simulink model "rising_hil"  (R2019b)
settings: Solver=FixedStepAuto  StartTime=0.0  StopTime=30  FixedStep=1  RelTol=1e-3
model workspace (MAT data in the model file):
  ALS_mode = Simulink.Signal
  ALS_mode.DataType = 'Enum: angle'
  ALS_mode.Dimensions = -1
  ALS_mode.DimensionsMode = 'auto'
  ALS_mode.Complexity = 'auto'
  ALS_mode.SampleTime = -1
  ALS_mode.SamplingMode = 'auto'
  ALS_mode_off = Simulink.Parameter
  ALS_mode_off.DataType = 'Enum: angle'
  ALS_mode_off.Dimensions = [0 0]
  ALS_mode_on = Simulink.Parameter
  ALS_mode_on.DataType = 'Enum: angle'
  ALS_mode_on.Dimensions = [0 0]
  Angle = Simulink.Signal
  Angle.DataType = 'uint8'
  Angle.Dimensions = -1
  Angle.DimensionsMode = 'auto'
  Angle.Complexity = 'auto'
  Angle.SampleTime = -1
  Angle.SamplingMode = 'auto'
  Carangle = Simulink.Parameter
  Carangle.Value = 25
  Carangle.DataType = 'uint8'
  Carangle.Dimensions = [1 1]
  Darkness_mode = Simulink.Signal
  Darkness_mode.DataType = 'Enum: angle'
  Darkness_mode.Dimensions = -1
  Darkness_mode.DimensionsMode = 'auto'
  Darkness_mode.Complexity = 'auto'
  Darkness_mode.SampleTime = -1
  Darkness_mode.SamplingMode = 'auto'
  Darkness_mode_off = Simulink.Parameter
  Darkness_mode_off.DataType = 'Enum: angle'
  Darkness_mode_off.Dimensions = [0 0]
  Darkness_mode_on = Simulink.Parameter
  Darkness_mode_on.DataType = 'Enum: angle'
  Darkness_mode_on.Dimensions = [0 0]
  Headlight_off = Simulink.Parameter
  Headlight_off.DataType = 'Enum: angle'
  Headlight_off.Dimensions = [0 0]
  High_Beam = Simulink.Parameter
  High_Beam.DataType = 'Enum: angle'
  High_Beam.Dimensions = [0 0]
  Ignition_off = Simulink.Parameter
  Ignition_off.DataType = 'angle'
  Ignition_off.Dimensions = [0 0]
  Ignition_on = Simulink.Parameter
  Ignition_on.DataType = 'Enum: angle'
  Ignition_on.Dimensions = [0 0]
  Ignitition = Simulink.Signal
  Ignitition.DataType = 'Enum:angle'
  Ignitition.Dimensions = -1
  Ignitition.DimensionsMode = 'auto'
  Ignitition.Complexity = 'auto'
  Ignitition.SampleTime = -1
  Ignitition.SamplingMode = 'auto'
  Low_Beam = Simulink.Parameter
  Low_Beam.DataType = 'Enum: angle'
  Low_Beam.Dimensions = [0 0]
  Time = Simulink.Parameter
  Time.Value = 2
  Time.DataType = 'uint8'
  Time.Dimensions = [1 1]
values from neighbouring files (symbols this model uses):
  Carangle = 25.0    [ALS_Project_dd.sldd]    (also in Car_Angle.m = Simulink.Parameter)
  Time = 2.0    [ALS_Project_dd.sldd]    (also in Car_Angle.m = Simulink.Parameter)
undefined symbols (not defined in the file or in its folder): angle, sigbuilder_block
libraries: simulink x6
settings Model: DataDictionary=Rising_hill_Data_Dictionary_2.sldd  OrderedModelArguments=off  Creator=Pravin  LastModifiedBy=Pravin
settings OptimizationCC: DefaultParameterBehavior=Inlined  EnhancedBackFolding=on  PassReuseOutputArgsAs=Individual arguments  ZeroExternalMemoryAtStartup=off  ZeroInternalMemoryAtStartup=off  OptimizeBlockOrder=speed  DifferentSizesBufferReuse=on  OptimizationCustomize=off  EfficientTunableParamExpr=on
settings DebuggingCC: ParameterTunabilityLossMsg=error
settings SFSimCC: MATLABDynamicMemAlloc=off
settings RTWCC: SystemTargetFile=ert.tlc  GenCodeOnly=on  TemplateMakefile=ert_default_tmf  GenerateReport=on  IncludeHyperlinkInReport=on  LaunchReport=on  GenerateTraceInfo=on  GenerateTraceReport=on  GenerateTraceReportSl=on  GenerateTraceReportSf=on  GenerateTraceReportEml=on
settings CodeAppCC: ForceParamTrailComments=on  IgnoreCustomStorageClasses=off  OperatorAnnotations=on  SimulinkDataObjDesc=on  SFDataObjDesc=on  InsertBlockDesc=on
settings ERTTargetCC: TargetLangStandard=C99 (ISO)  GenerateSampleERTMain=on  InlinedParameterPlacement=NonHierarchical  ERTCustomFileTemplate=example_file_process.tlc
settings ConfigComp: CovMetricSettings=dcmwe

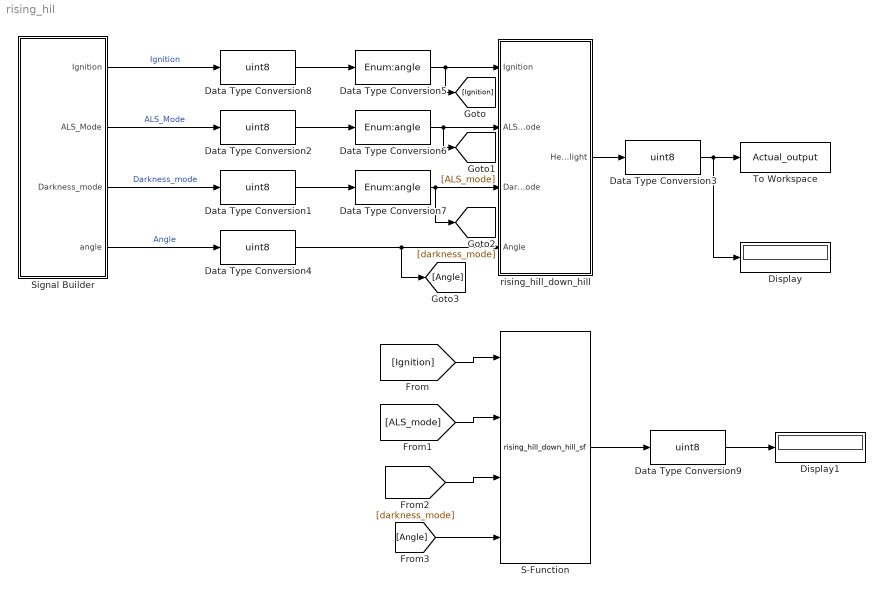
== system rising_hil ==
  Data Type Conversion{1..2,4,8} (4 alike) : DataTypeConversion  OutDataTypeStr=uint8  SaturateOnIntegerOverflow=on
  Data Type Conversion3 : DataTypeConversion  OutDataTypeStr=uint8
  Data Type Conversion5 : DataTypeConversion  OutDataTypeStr=Enum:angle  SaturateOnIntegerOverflow=on
  Data Type Conversion6 : DataTypeConversion  OutDataTypeStr=Enum:angle  SaturateOnIntegerOverflow=on
  Data Type Conversion7 : DataTypeConversion  OutDataTypeStr=Enum:angle  SaturateOnIntegerOverflow=on
  Data Type Conversion9 : DataTypeConversion  OutDataTypeStr=uint8
  Display : Display
  Display1 : Display
  S-Function : S-Function  FunctionName=rising_hill_down_hill_sf  SFunctionDeploymentMode=off  EnableBusSupport=off  SFcnStateName=DWORK0
      settings: SFcnIsStateOwnerBlock=on
  Signal Builder : Subsystem  Tag=STV Subsys  LoadFcn=sigbuilder_block('load',[437.6 153 550.4 359.25 ]);  StartFcn=sigbuilder_block('start');  StopFcn=sigbuilder_block('stop');  ClipboardFcn=sigbuilder_block('clipboard');  mask(Sigbuilder block){tuvar=[0:10]}
      mask help: Simulink:masks:SigbuilderBlock_MD
      mask init:
      | if ~strcmp(get_param(bdroot(gcbh),'SimulationStatus'),'stopped') tuvar = sigbuilder_block('maskInit'); end
      settings: CopyFcn=sigbuilder_block('copy');  DeleteFcn=sigbuilder_block('delete');  ModelCloseFcn=sigbuilder_block('modelClose');  PreSaveFcn=sigbuilder_block('preSave');  PauseFcn=sigbuilder_block('pause');  ContinueFcn=sigbuilder_block('continue');  NameChangeFcn=sigbuilder_block('namechange');  OpenFcn=sigbuilder_block('open',[437.6 153 550.4 359.25 ]);  CloseFcn=sigbuilder_block('close');
      mask Display: plot(0, 0, 100, 100,[2, 2, 32, 32, 2], [68, 8, 8, 68, 68],[32, 2], [38, 38], [32, 19, 2],[53, 60, 44], [32, 17, 17, 2],[16, 16, 31, 31]);txt = getActiveGroup(gcbh);text(2, 100, txt,'verticalAlignment', 'top');
  To Workspace : ToWorkspace  VariableName=Actual_output  SaveFormat=Timeseries  SampleTime=-1
  rising_hill_down_hill : Subsystem  TreatAsAtomicUnit=on
  wires:
  Signal Builder/4(angle) -> Data Type Conversion4/1  "Angle"
  rising_hill_down_hill/1("Headlight ") -> Data Type Conversion3/1
  Signal Builder/3(Darkness_mode) -> Data Type Conversion1/1  "Darkness_mode"
  Signal Builder/1(Ignition) -> Data Type Conversion8/1  "Ignition"
  Data Type Conversion5/1 -> [Ignition], rising_hill_down_hill/1(Ignition)
  Data Type Conversion6/1 -> rising_hill_down_hill/2("ALS_mode "), [ALS_mode]
  Data Type Conversion3/1 -> Display/1, To Workspace/1
  Data Type Conversion4/1 -> rising_hill_down_hill/4("Angle "), [Angle]
  Data Type Conversion7/1 -> rising_hill_down_hill/3("Darkness_mode "), [darkness_mode]
  Signal Builder/2(ALS_Mode) -> Data Type Conversion2/1  "ALS_Mode"
  Data Type Conversion1/1 -> Data Type Conversion7/1
  Data Type Conversion2/1 -> Data Type Conversion6/1
  Data Type Conversion8/1 -> Data Type Conversion5/1
  [Ignition] -> S-Function/1
  [ALS_mode] -> S-Function/2
  [darkness_mode] -> S-Function/3
  [Angle] -> S-Function/4
  S-Function/1 -> Data Type Conversion9/1
  Data Type Conversion9/1 -> Display1/1

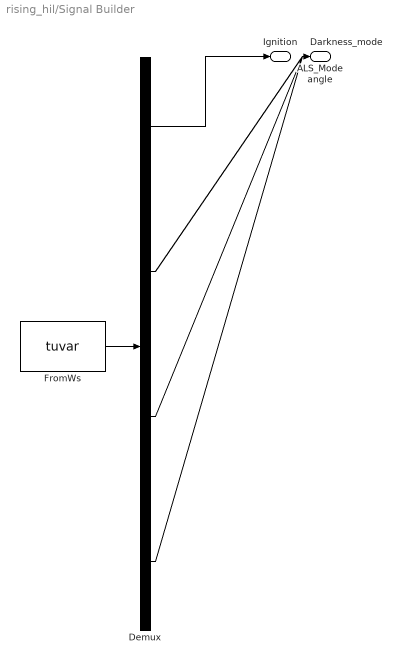
== system rising_hil/Signal Builder ==
  Demux : Demux  Tag=STV Demux
  FromWs : FromWorkspace  Tag=STV FromWs  VariableName=tuvar  SampleTime=0
      SigBuilderData=|
      | common.afterFinalStr = 'Extrapolate'
      | common.sampleTime = 0
      | dataSet.timeRange = [0 10]
      | dataSet.name = 'Sheet1'
      | sbobj.Name = 'Signal Builder'
      | sbobj.Groups.Name = 'Sheet1'
      | sbobj.Groups.Signals(1).Name = 'Ignition'
      | sbobj.Groups.Signals(1).XData = [0 1 2 3 4 5 6 7 8 9 10]
      | sbobj.Groups.Signals(1).YData = [2 3 2 2 2 2 3 3 2 2 2]
      | sbobj.Groups.Signals(2).Name = 'ALS_Mode'
      | sbobj.Groups.Signals(2).XData = [0 1 2 3 4 5 6 7 8 9 10]
      | sbobj.Groups.Signals(2).YData = [4 4 5 4 4 4 5 5 4 4 4]
      | sbobj.Groups.Signals(3).Name = 'Darkness_mode'
      | sbobj.Groups.Signals(3).XData = [0 1 2 3 4 5 6 7 8 9 10]
      | sbobj.Groups.Signals(3).YData = [6 6 6 7 6 6 7 7 6 6 6]
      | sbobj.Groups.Signals(4).Name = 'angle'
      | sbobj.Groups.Signals(4).XData = [0 1 2 3 4 5 6 7 8 9 10]
      | sbobj.Groups.Signals(4).YData = [20 25 26 25 25 25 20 26 26 22 0]
  Ignition : Outport  Tag=STV Outport
  ALS_Mode : Outport  Tag=STV Outport  Port=2
  Darkness_mode : Outport  Tag=STV Outport  Port=3
  angle : Outport  Tag=STV Outport  Port=4
  wires:
  Demux/1 -> Ignition/1
  FromWs/1 -> Demux/1
  Demux/2 -> ALS_Mode/1
  Demux/3 -> Darkness_mode/1
  Demux/4 -> angle/1

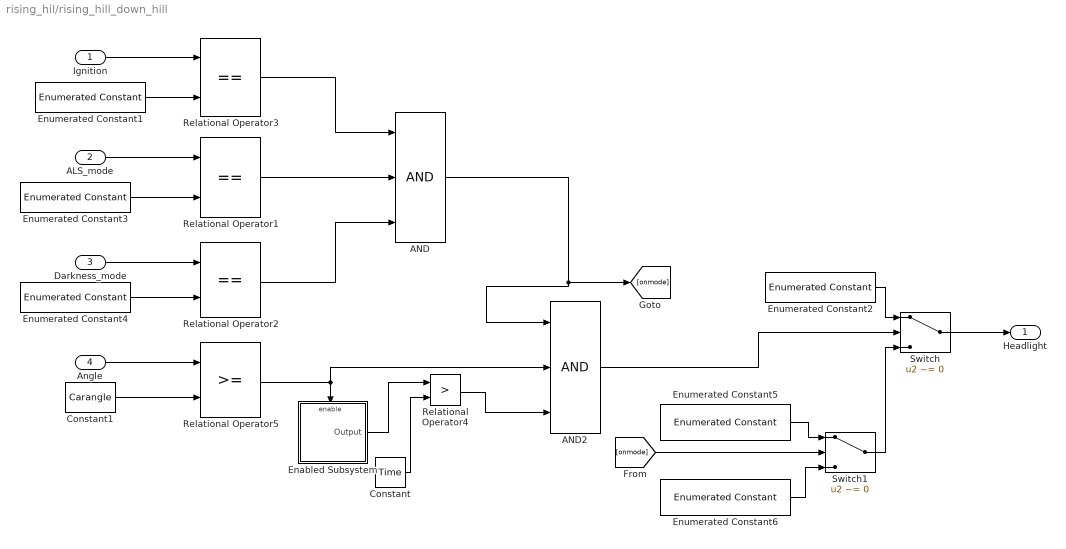
== system rising_hil/rising_hill_down_hill ==
  Ignition : Inport
  "ALS_mode " : Inport  Port=2
  "Darkness_mode " : Inport  Port=3
  "Angle " : Inport  Port=4
  AND : Logic  Inputs=3  AllPortsSameDT=off  OutDataTypeStr=boolean
  AND2 : Logic  Inputs=3  AllPortsSameDT=off  OutDataTypeStr=boolean
  Constant : Constant  Value=Time
  Constant1 : Constant  Value=Carangle
  Enabled Subsystem : Subsystem  TreatAsAtomicUnit=on
  Enumerated Constant1 : simulink/Sources/Enumerated Constant  OutDataTypeStr=Enum:angle  Value=angle.Ignition_on  SampleTime=inf
      settings: SourceProductName=Simulink
  Enumerated Constant2 : simulink/Sources/Enumerated Constant  OutDataTypeStr=Enum:angle  Value=angle.High_Beam  SampleTime=inf
      settings: SourceProductName=Simulink
  Enumerated Constant3 : simulink/Sources/Enumerated Constant  OutDataTypeStr=Enum:angle  Value=angle.ALS_mode_on  SampleTime=inf
      settings: SourceProductName=Simulink
  Enumerated Constant4 : simulink/Sources/Enumerated Constant  OutDataTypeStr=Enum:angle  Value=angle.Darkness_mode_on  SampleTime=inf
      settings: SourceProductName=Simulink
  Enumerated Constant5 : simulink/Sources/Enumerated Constant  OutDataTypeStr=Enum:angle  Value=angle.Low_Beam  SampleTime=inf
      settings: SourceProductName=Simulink
  Enumerated Constant6 : simulink/Sources/Enumerated Constant  OutDataTypeStr=Enum:angle  Value=angle.Headlight_off  SampleTime=inf
      settings: SourceProductName=Simulink
  Relational Operator1 : RelationalOperator  Operator===  OutDataTypeStr=boolean  RndMeth=Simplest
  Relational Operator2 : RelationalOperator  Operator===  OutDataTypeStr=boolean  RndMeth=Simplest
  Relational Operator3 : RelationalOperator  Operator===  OutDataTypeStr=boolean  RndMeth=Simplest
  Relational Operator4 : RelationalOperator  Operator=>  OutDataTypeStr=boolean  RndMeth=Simplest
  Relational Operator5 : RelationalOperator  OutDataTypeStr=boolean  RndMeth=Simplest
  Switch : Switch  Criteria=u2 ~= 0
  Switch1 : Switch  Criteria=u2 ~= 0
  "Headlight " : Outport
  wires:
  "Darkness_mode "/1 -> Relational Operator2/1
  Enumerated Constant4/1 -> Relational Operator2/2
  Enumerated Constant3/1 -> Relational Operator1/2
  "ALS_mode "/1 -> Relational Operator1/1
  Ignition/1 -> Relational Operator3/1
  Enumerated Constant1/1 -> Relational Operator3/2
  AND/1 -> AND2/1, [onmode]
  Enabled Subsystem/1(Output) -> Relational Operator4/1
  Constant/1 -> Relational Operator4/2
  Relational Operator5/1 -> AND2/2, Enabled Subsystem/Enable
  Switch1/1 -> Switch/3
  Switch/1 -> "Headlight "/1
  Enumerated Constant6/1 -> Switch1/3
  Enumerated Constant2/1 -> Switch/1
  Enumerated Constant5/1 -> Switch1/1
  Relational Operator1/1 -> AND/2
  Relational Operator2/1 -> AND/3
  Relational Operator3/1 -> AND/1
  [onmode] -> Switch1/2
  AND2/1 -> Switch/2
  "Angle "/1 -> Relational Operator5/1
  Constant1/1 -> Relational Operator5/2
  Relational Operator4/1 -> AND2/3

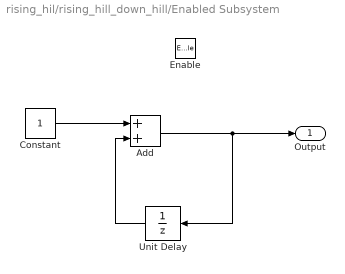
== system rising_hil/rising_hill_down_hill/Enabled Subsystem ==
  Enable : EnablePort  StatesWhenEnabling=reset
  Add : Sum
  Constant : Constant
  Unit Delay : UnitDelay  SampleTime=-1  HasFrameUpgradeWarning=on
  Output : Outport  OutputWhenDisabled=reset  InitialOutput=[0]
  wires:
  Constant/1 -> Add/1
  Add/1 -> Unit Delay/1, Output/1
  Unit Delay/1 -> Add/2
